simulink model "motorv1_2(1)"  (R2024a)
settings: Solver=VariableStepAuto  StartTime=0.0  StopTime=0.02  RelTol=1e-3
undefined symbols (not defined in the file): DiscIntNeverNeededParam, sigbuilder_block, Ts
libraries: spsUniversalBridgeLib x2, spsCurrentMeasurementLib x2, spsControlledCurrentSourceLib x2, spsVoltageMeasurementLib x2, spsDCVoltageSourceLib x1, spspowerguiLib x1
settings Model: Creator=杨帅  LastModifiedBy=One
settings ModelReferenceCC: EnableRefExpFcnMdlSchedulingChecks=on
settings RTWCC: GPUComputeCapability=3.5

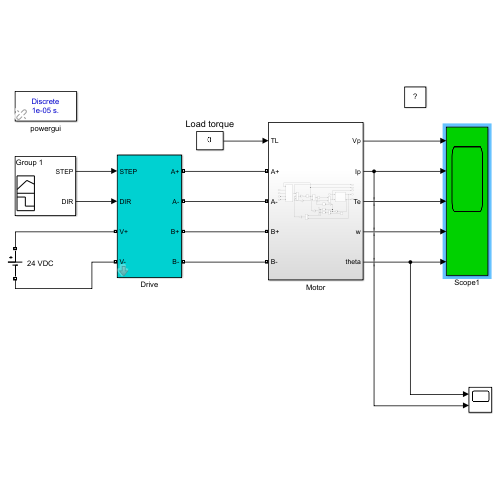
[thumbnail: Simulink's stored preview of the top-level diagram]
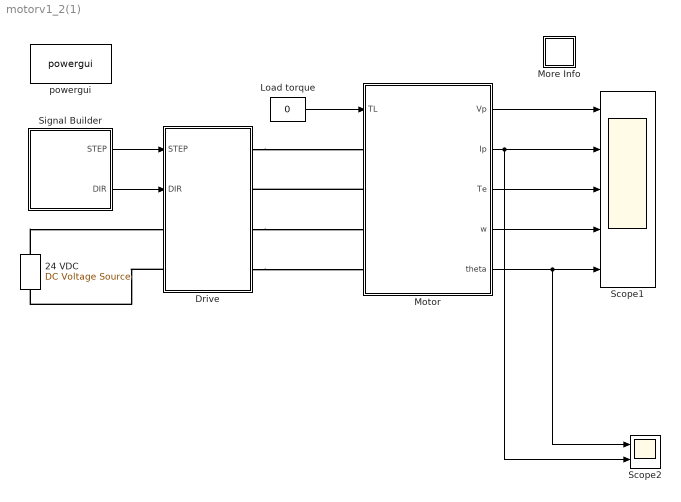
== system motorv1_2(1) ==
  24 VDC : spsDCVoltageSourceLib/DC Voltage Source  Amplitude=24  Measurements=None
  Drive : Subsystem  mask{Iref=2, step=500, Ts=Ts}
      mask prompts: Iref "Phase current (A)"; step "Stepping rate (step/s)"; Ts "Sampling time (s)"
      mask init:
      | Nstep=round(1/step/Ts);
  Load torque : Constant  Value=0
  More Info : Subsystem
      settings: OpenFcn=showdemo(bdroot(gcb))
      mask Display: disp('?')
  Motor : Subsystem
  Scope1 : Scope  NumInputPorts=5
  Scope2 : Scope  NumInputPorts=2
  Signal Builder : Subsystem  Tag=STV Subsys  LoadFcn=sigbuilder_block('load');  StartFcn=sigbuilder_block('start');  StopFcn=sigbuilder_block('stop');  ClipboardFcn=sigbuilder_block('clipboard');  mask(Sigbuilder block){tuvar=[0:10]}
      mask help: Sigbuilder GUI
      mask init:
      | if ~strcmp(get_param(bdroot(gcbh),'SimulationStatus'),'stopped') tuvar = sigbuilder_block('maskInit'); end
      settings: CopyFcn=sigbuilder_block('copy');  DeleteFcn=sigbuilder_block('delete');  ModelCloseFcn=sigbuilder_block('modelClose');  PreSaveFcn=sigbuilder_block('preSave');  PauseFcn=sigbuilder_block('pause')  ContinueFcn=sigbuilder_block('continue')  NameChangeFcn=sigbuilder_block('namechange');  OpenFcn=sigbuilder_block('open',[162.75 86 550.5 364 ]);  CloseFcn=sigbuilder_block('close');
      mask Display: plot(0, 0, 100, 100,[2, 2, 32, 32, 2], [68, 8, 8, 68, 68],[32, 2], [38, 38], [32, 19, 2],[53, 60, 44], [32, 17, 17, 2],[16, 16, 31, 31]);txt = getActiveGroup(gcbh);text(2, 100, txt,'verticalAlignment', 'top');
  powergui : spspowerguiLib/powergui  Priority=1  SimulationMode=Discrete  SampleTime=10e-6  frequency=60  Iterations=50  frequencyindice=0  Pbase=100e6  ErrMax=1e-4  UnitsV=kV  UnitsW=MW  buscounter=0  FunctionMessages=off  echomessages=off  EnableUseOfTLC=off  CurrentSourceSwitches=off  DisableSnubberDevices=off  DisableRonSwitches=off  DisableVfSwitches=off  DisplayEquations=off  AutomaticDiscreteSolvers=off  SolverType=Tustin/Backward Euler (TBE)  Interpol=off  ExternalGateDelay=off  methode=off  Ts=100  x0status=blocks  SPID=on  SwTol=0  HookPort=off  NonlinearTolerance=1e-4  nMaxIteration=100  ContinueOnMaxIteration=off  RestoreLinks=warning  ResistiveCurrentMeasurement=off  Frange=[0:2:500]  Ylog=off  Xlog=on  ShowGrid=off  save=off  variable=ZData  structure=0  ZoomFFT=off  StartTime=0.0  cycles=1  DisplayStyle=1  fundamental=60  FreqAxis=off  MaxFrequency=1000  frequencyindicesteady=1  RmsSteady=1  display=off
  wires:
  Signal Builder/1(STEP) -> Drive/1(STEP)
  Signal Builder/2(DIR) -> Drive/2(DIR)
  Load torque/1 -> Motor/1(TL)
  Motor/1(Vp) -> Scope1/1
  Motor/2(Ip) -> Scope2/2, Scope1/2
  Motor/3(Te) -> Scope1/3
  Motor/4(w) -> Scope1/4
  Motor/5(theta) -> Scope2/1, Scope1/5
  connections:
  Drive/RConn4 -- Motor/LConn4
  Motor/LConn2 -- Drive/RConn2
  Drive/RConn1 -- Motor/LConn1
  24 VDC/RConn1 -- Drive/LConn1
  Drive/LConn2 -- 24 VDC/LConn1
  Drive/RConn3 -- Motor/LConn3

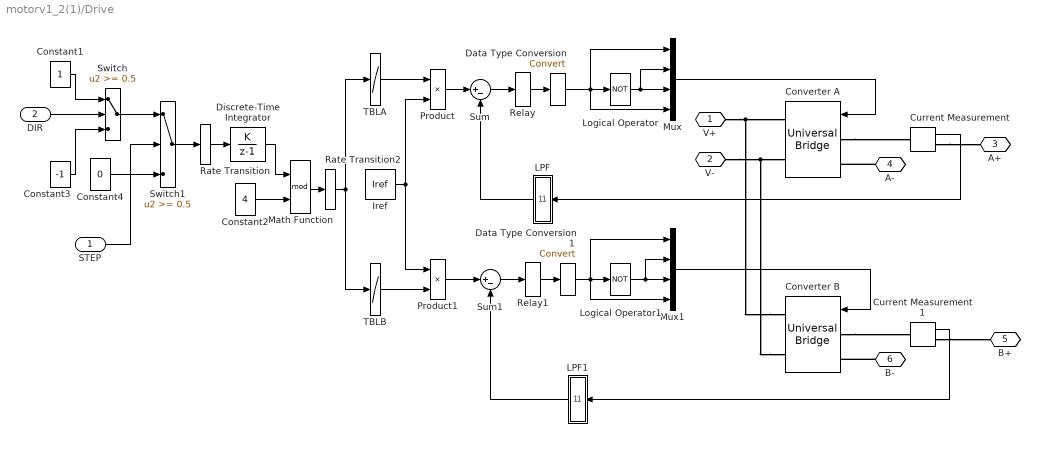
== system motorv1_2(1)/Drive ==
  STEP : Inport
  DIR : Inport  Port=2
  Constant1 : Constant  SampleTime=Ts
  Constant2 : Constant  Value=4  SampleTime=Nstep*Ts
  Constant3 : Constant  Value=-1  SampleTime=Ts
  Constant4 : Constant  Value=0  SampleTime=Ts
  Converter A : spsUniversalBridgeLib/Universal Bridge  Arms=2  SnubberResistance=10000  SnubberCapacitance=inf  Device=MOSFET / Diodes  Ron=1e-3*10  Lon=0  ForwardVoltages="[  0  0  ]"  ForwardVoltage=0  GTOparameters=[ 10e-6 , 20e-6 ]  IGBTparameters=[ 0.5e-6 , 0.5e-6 ]  Measurements=None  Measurements_2=None  converterType=Rectifier
  Converter B : spsUniversalBridgeLib/Universal Bridge  Arms=2  SnubberResistance=10000  SnubberCapacitance=inf  Device=MOSFET / Diodes  Ron=1e-3*10  Lon=0  ForwardVoltages="[  0  0  ]"  ForwardVoltage=0  GTOparameters=[ 10e-6 , 20e-6 ]  IGBTparameters=[ 0.5e-6 , 0.5e-6 ]  Measurements=None  Measurements_2=None  converterType=Rectifier
  Current Measurement : spsCurrentMeasurementLib/Current Measurement  PhasorSimulation=off  OutputType=Complex  PSBequivalent=0
  Current Measurement1 : spsCurrentMeasurementLib/Current Measurement  PhasorSimulation=off  OutputType=Complex  PSBequivalent=0
  Data Type Conversion : DataTypeConversion  SaturateOnIntegerOverflow=off  RndMeth=Floor
  Data Type Conversion1 : DataTypeConversion  SaturateOnIntegerOverflow=off  RndMeth=Floor
  Discrete-Time Integrator : DiscreteIntegrator  IntegratorMethod=Accumulation: Forward Euler  SampleTime=Nstep*Ts  ICPrevOutput=DiscIntNeverNeededParam  ICPrevScaledInput=DiscIntNeverNeededParam
  Iref : Constant  Value=Iref  SampleTime=Ts
  LPF : Subsystem  mask{fc=10000, Ts=Ts}
      mask prompts: fc "Cut-off frequency (Hz)"; Ts "Sampling time (s)"
      mask init:
      | % fa=tf(1,[1/2/pi/fc 1]);
      | % fn=c2d(fa,Ts);
      | % [NN,DD]=tfdata(fn,'v')
      | 
      | NN = [ 0,0.0609];
      | DD = [1.0000,-0.9391];
  LPF1 : Subsystem  mask{fc=10000, Ts=Ts}
      mask prompts: fc "Cut-off frequency (Hz)"; Ts "Sampling time (s)"
      mask init:
      | % fa=tf(1,[1/2/pi/fc 1]);
      | % fn=c2d(fa,Ts);
      | % [NN,DD]=tfdata(fn,'v')
      | 
      | NN = [ 0,0.0609];
      | DD = [1.0000,-0.9391];
  Logical Operator : Logic  Operator=NOT  AllPortsSameDT=off  OutDataTypeStr=boolean
  Logical Operator1 : Logic  Operator=NOT  AllPortsSameDT=off  OutDataTypeStr=boolean
  Math Function : Math  Operator=mod  SignedPower=on  SampleTime=Nstep*Ts
  Mux : Mux
  Mux1 : Mux
  Product : Product  RndMeth=Zero
  Product1 : Product  RndMeth=Zero
  Rate Transition : RateTransition
  Rate Transition2 : RateTransition
  Relay : Relay  OnSwitchValue=0.01  OffSwitchValue=-0.01
  Relay1 : Relay  OnSwitchValue=0.01  OffSwitchValue=-0.01  OutDataTypeStr=Inherit: Inherit via back propagation
  Sum : Sum  Inputs=|+-  OutDataTypeStr=Inherit: Same as first input
  Sum1 : Sum  Inputs=|+-  OutDataTypeStr=Inherit: Same as first input
  Switch : Switch  Threshold=0.5  ZeroCross=off  SampleTime=Ts  SaturateOnIntegerOverflow=off  InputSameDT=off
  Switch1 : Switch  Threshold=0.5  ZeroCross=off  SampleTime=Ts  SaturateOnIntegerOverflow=off  InputSameDT=off
  TBLA : Lookup_n-D  NumberOfTableDimensions=1  BreakpointsForDimension1=[0:3]  BreakpointsForDimension2=[0 571.55 685.8 800.15 914.4 1028.8 1143.1 1257.4 1371.7 1486 1600.3 1714.6 1828.9 1943.2 2057.5 2171.8 2286.1 2400.5 2514.7 2629.1 2743.3 2857.7 2971.9 3086.3 3200.5 3314.9 3429.2]  Table=[1 0 -1 0]  InternalRulePriority=Speed  RndMeth=Simplest
  TBLB : Lookup_n-D  NumberOfTableDimensions=1  BreakpointsForDimension1=[0:3]  BreakpointsForDimension2=[0 571.55 685.8 800.15 914.4 1028.8 1143.1 1257.4 1371.7 1486 1600.3 1714.6 1828.9 1943.2 2057.5 2171.8 2286.1 2400.5 2514.7 2629.1 2743.3 2857.7 2971.9 3086.3 3200.5 3314.9 3429.2]  Table=[0 1 0 -1]  InternalRulePriority=Speed  RndMeth=Simplest
  V+ : PMIOPort  Side=Left
  V- : PMIOPort  Port=2  Side=Left
  A+ : PMIOPort  Port=3  Side=Right
  A- : PMIOPort  Port=4  Side=Right
  B+ : PMIOPort  Port=5  Side=Right
  B- : PMIOPort  Port=6  Side=Right
  wires:
  Constant4/1 -> Switch1/3
  Switch1/1 -> Rate Transition/1
  Switch/1 -> Switch1/1
  STEP/1 -> Switch1/2
  DIR/1 -> Switch/2
  Rate Transition2/1 -> TBLB/1, TBLA/1
  Math Function/1 -> Rate Transition2/1
  Product1/1 -> Sum1/1
  Product/1 -> Sum/1
  Rate Transition/1 -> Discrete-Time Integrator/1
  Constant3/1 -> Switch/3
  Constant1/1 -> Switch/1
  Discrete-Time Integrator/1 -> Math Function/1
  Constant2/1 -> Math Function/2
  Iref/1 -> Product1/1, Product/2
  TBLB/1 -> Product1/2
  TBLA/1 -> Product/1
  LPF1/1(O) -> Sum1/2
  LPF/1(O) -> Sum/2
  Data Type Conversion1/1 -> Mux1/4, Mux1/1, Logical Operator1/1
  Data Type Conversion/1 -> Logical Operator/1, Mux/4, Mux/1
  Current Measurement1/1 -> LPF1/1(I)
  Sum1/1 -> Relay1/1
  Mux1/1 -> Converter B/1
  Logical Operator1/1 -> Mux1/2, Mux1/3
  Relay1/1 -> Data Type Conversion1/1
  Mux/1 -> Converter A/1
  Logical Operator/1 -> Mux/2, Mux/3
  Relay/1 -> Data Type Conversion/1
  Current Measurement/1 -> LPF/1(I)
  Sum/1 -> Relay/1
  connections:
  Converter B/RConn2 -- Converter A/RConn2 -- V-/RConn1
  Converter B/RConn1 -- Converter A/RConn1 -- V+/RConn1
  Current Measurement1/RConn1 -- B+/RConn1
  Converter B/LConn1 -- Current Measurement1/LConn1
  Current Measurement/RConn1 -- A+/RConn1
  Converter A/LConn1 -- Current Measurement/LConn1
  B-/RConn1 -- Converter B/LConn2
  A-/RConn1 -- Converter A/LConn2

== system motorv1_2(1)/More Info ==

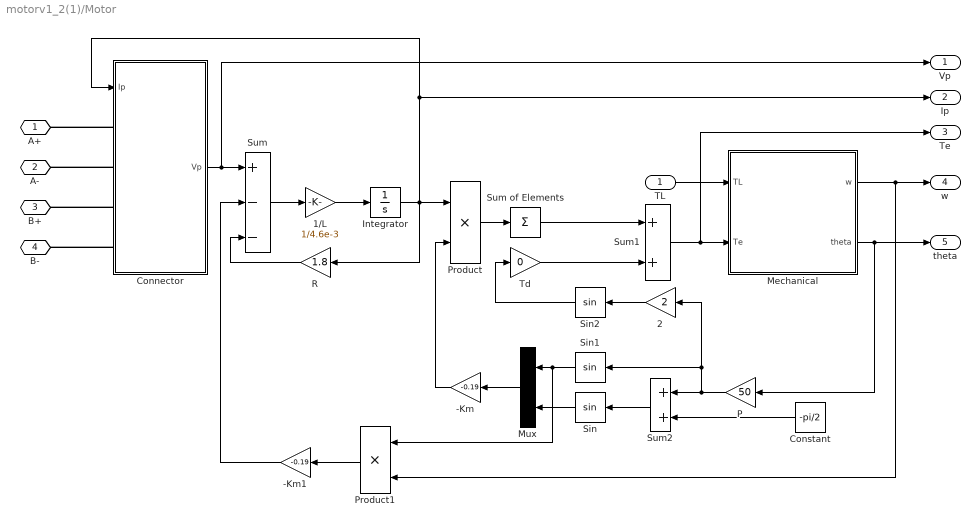
== system motorv1_2(1)/Motor ==
  TL : Inport
  -Km : Gain  Gain=-0.19
  -Km1 : Gain  Gain=-0.19
  1/L : Gain  Gain=1/4.6e-3
  2 : Gain  Gain=2
  Connector : Subsystem
  Constant : Constant  Value=-pi/2
  Integrator : Integrator
  Mechanical : Subsystem
  Mux : Mux  Inputs=2
  P : Gain  Gain=50
  Product : Product
  Product1 : Product
  R : Gain  Gain=1.8
  Sin : Trigonometry
  Sin1 : Trigonometry
  Sin2 : Trigonometry
  Sum : Sum  Inputs=+--
  Sum of Elements : Sum  Inputs=+
  Sum1 : Sum
  Sum2 : Sum
  Td : Gain  Gain=0
  A+ : PMIOPort  Side=Left
  A- : PMIOPort  Port=2  Side=Left
  B+ : PMIOPort  Port=3  Side=Left
  B- : PMIOPort  Port=4  Side=Left
  Vp : Outport
  Ip : Outport  Port=2
  Te : Outport  Port=3
  w : Outport  Port=4
  theta : Outport  Port=5
  wires:
  -Km/1 -> Product/2
  Sum/1 -> 1/L/1
  P/1 -> 2/1, Sin1/1, Sum2/1
  1/L/1 -> Integrator/1
  Mechanical/2(theta) -> theta/1, P/1
  Mechanical/1(w) -> Product1/2, w/1
  Product/1 -> Sum of Elements/1
  -Km1/1 -> Sum/2
  Sin2/1 -> Td/1
  Td/1 -> Sum1/2
  Sin1/1 -> Product1/1, Mux/1
  2/1 -> Sin2/1
  Integrator/1 -> Product/1, Ip/1, Connector/1(Ip), R/1
  Constant/1 -> Sum2/2
  Sum of Elements/1 -> Sum1/1
  Connector/1(Vp) -> Vp/1, Sum/1
  R/1 -> Sum/3
  Mux/1 -> -Km/1
  Sin/1 -> Mux/2
  Sum2/1 -> Sin/1
  Product1/1 -> -Km1/1
  Sum1/1 -> Te/1, Mechanical/2(Te)
  TL/1 -> Mechanical/1(TL)
  connections:
  Connector/LConn4 -- B-/RConn1
  Connector/LConn3 -- B+/RConn1
  Connector/LConn2 -- A-/RConn1
  Connector/LConn1 -- A+/RConn1

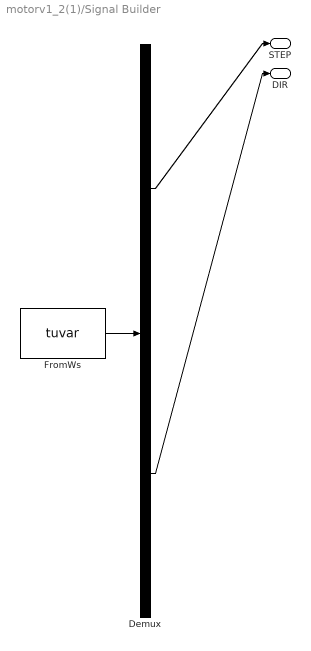
== system motorv1_2(1)/Signal Builder ==
  Demux : Demux  Tag=STV Demux  Outputs=2
      settings: DisplayOption=none
  FromWs : FromWorkspace  Tag=STV FromWs  VariableName=tuvar
      SigBuilderData=|
      | common.afterFinalStr = 'Extrapolate'
      | common.sampleTime = 0
      | dataSet.timeRange = [0 0.25]
      | dataSet.name = 'Group 1'
      | sbobj.Groups.Name = 'Group 1'
      | sbobj.Groups.Signals(1).Name = 'STEP'
      | sbobj.Groups.Signals(1).XData = [0 0.1 0.10001 0.15 0.15001 0.2 0.20001 0.25]
      | sbobj.Groups.Signals(1).YData = [1 1 0 0 1 1 0 0]
      | sbobj.Groups.Signals(2).Name = 'DIR'
      | sbobj.Groups.Signals(2).XData = [0 0.1 0.10001 0.25]
      | sbobj.Groups.Signals(2).YData = [1 1 0 0]
      | sbobj.Groups.TimeRange = [0 0.25]
  STEP : Outport  Tag=STV Outport  VectorParamsAs1DForOutWhenUnconnected=off
  DIR : Outport  Tag=STV Outport  Port=2  VectorParamsAs1DForOutWhenUnconnected=off
  wires:
  FromWs/1 -> Demux/1
  Demux/1 -> STEP/1
  Demux/2 -> DIR/1

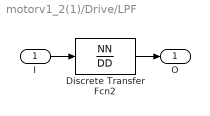
== system motorv1_2(1)/Drive/LPF ==
  I : Inport
  Discrete Transfer Fcn2 : DiscreteTransferFcn  Numerator=NN  Denominator=DD  SampleTime=Ts
  O : Outport  VectorParamsAs1DForOutWhenUnconnected=off
  wires:
  Discrete Transfer Fcn2/1 -> O/1
  I/1 -> Discrete Transfer Fcn2/1

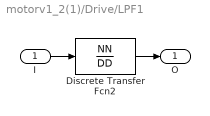
== system motorv1_2(1)/Drive/LPF1 ==
  I : Inport
  Discrete Transfer Fcn2 : DiscreteTransferFcn  Numerator=NN  Denominator=DD  SampleTime=Ts
  O : Outport  VectorParamsAs1DForOutWhenUnconnected=off
  wires:
  I/1 -> Discrete Transfer Fcn2/1
  Discrete Transfer Fcn2/1 -> O/1

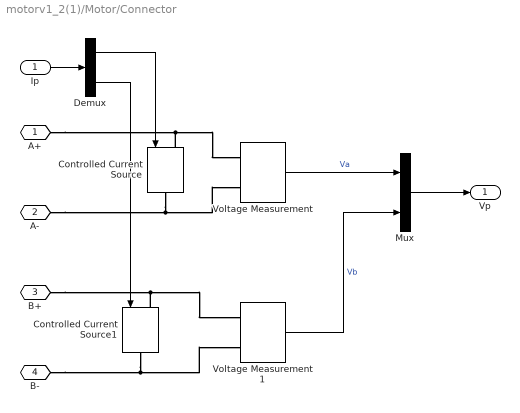
== system motorv1_2(1)/Motor/Connector ==
  Ip : Inport
  Controlled Current Source : spsControlledCurrentSourceLib/Controlled Current Source  Initialize=on  Source_Type=DC  Amplitude=2  Phase=0  Frequency=0  Measurements=None
  Controlled Current Source1 : spsControlledCurrentSourceLib/Controlled Current Source  Initialize=on  Source_Type=DC  Amplitude=2  Phase=0  Frequency=0  Measurements=None
  Demux : Demux  Outputs=2
  Mux : Mux  Inputs=2
  Voltage Measurement : spsVoltageMeasurementLib/Voltage Measurement  PhasorSimulation=off  OutputType=Complex  PSBequivalent=0
  Voltage Measurement1 : spsVoltageMeasurementLib/Voltage Measurement  PhasorSimulation=off  OutputType=Complex  PSBequivalent=0
  A+ : PMIOPort  Side=Left
  A- : PMIOPort  Port=2  Side=Left
  B+ : PMIOPort  Port=3  Side=Left
  B- : PMIOPort  Port=4  Side=Left
  Vp : Outport
  wires:
  Mux/1 -> Vp/1
  Ip/1 -> Demux/1
  Demux/1 -> Controlled Current Source/1
  Demux/2 -> Controlled Current Source1/1
  Voltage Measurement/1 -> Mux/1  "Va"
  Voltage Measurement1/1 -> Mux/2  "Vb"
  connections:
  A+/RConn1 -- Controlled Current Source/LConn1 -- Voltage Measurement/LConn1
  A-/RConn1 -- Controlled Current Source/RConn1 -- Voltage Measurement/LConn2
  B+/RConn1 -- Voltage Measurement1/LConn1 -- Controlled Current Source1/LConn1
  B-/RConn1 -- Controlled Current Source1/RConn1 -- Voltage Measurement1/LConn2

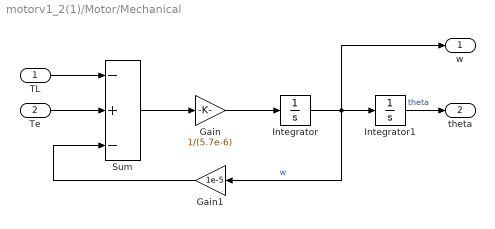
== system motorv1_2(1)/Motor/Mechanical ==
  TL : Inport
  Te : Inport  Port=2
  Gain : Gain  Gain=1/(5.7e-6)
  Gain1 : Gain  Gain=1e-5
  Integrator : Integrator
  Integrator1 : Integrator
  Sum : Sum  Inputs=-+-
  w : Outport
  theta : Outport  Port=2
  wires:
  Te/1 -> Sum/2
  TL/1 -> Sum/1
  Sum/1 -> Gain/1
  Gain/1 -> Integrator/1
  Integrator/1 -> Gain1/1, w/1, Integrator1/1  "w"
  Integrator1/1 -> theta/1  "theta"
  Gain1/1 -> Sum/3
